simulink model "exp3"  (R2021b)
settings: Solver=VariableStepAuto  StartTime=0.0  StopTime=10.0  RelTol=1e-3
settings Model: Creator=ashir  LastModifiedBy=ashir

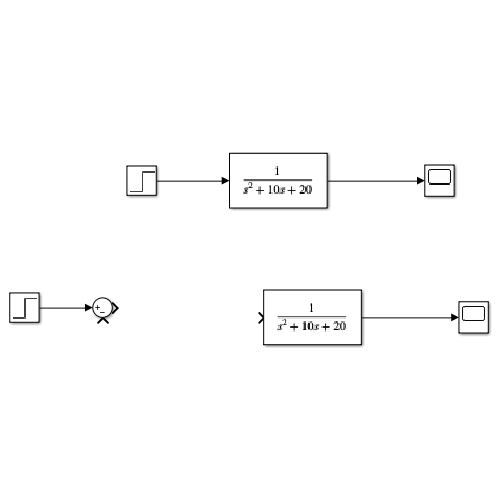
[thumbnail: Simulink's stored preview of the top-level diagram]
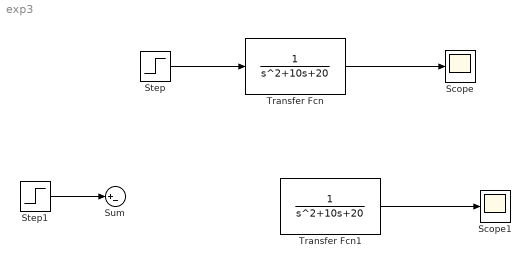
== system exp3 ==
  Scope : Scope
  Scope1 : Scope
  Step : Step  Time=0  SampleTime=0
  Step1 : Step  Time=0  SampleTime=0
  Sum : Sum  Inputs=|+-
  Transfer Fcn : TransferFcn  Denominator=[1 10 20]
  Transfer Fcn1 : TransferFcn  Denominator=[1 10 20]
  wires:
  Transfer Fcn/1 -> Scope/1
  Step/1 -> Transfer Fcn/1
  Transfer Fcn1/1 -> Scope1/1
  Step1/1 -> Sum/1
